simulink library "alphaBetaLE_ul"  (R2020a)
settings: Solver=VariableStepAuto  StartTime=0.0  StopTime=10.0  RelTol=1e-3
libraries: vrlib x1, vectorNormalizer_ul x1
settings Model: Creator=mcobb  LastModifiedBy=John Jr
settings DataIOCC: ReturnWorkspaceOutputs=off
settings DebuggingCC: ArithmeticOperatorsInVariantConditions=warning
settings SFSimCC: CustomCodeUndefinedFunction=UseInterfaceOnly

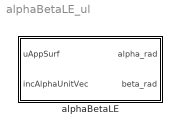
== system alphaBetaLE_ul ==
  alphaBetaLE : Subsystem  TreatAsAtomicUnit=on
      settings: MinAlgLoopOccurrences=on

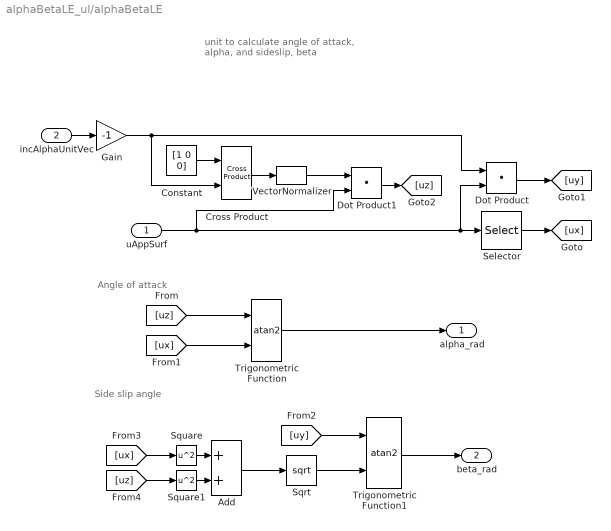
== system alphaBetaLE_ul/alphaBetaLE ==
  note: Side slip angle
  note: Angle of attack
  note: unit to calculate angle of attack,
      | alpha, and sideslip, beta
  uAppSurf : Inport
  incAlphaUnitVec : Inport  Port=2
  Add : Sum
  Constant : Constant  Value=[1 0 0]
  Cross Product : vrlib/Utilities/Cross Product
  Dot Product : DotProduct  InputSameDT=on  OutDataTypeStr=Inherit: Inherit via internal rule
  Dot Product1 : DotProduct  InputSameDT=on  OutDataTypeStr=Inherit: Inherit via internal rule
  Gain : Gain  Gain=-1
  Selector : Selector  InputPortWidth=3  IndexOptions=Index vector (dialog)  Indices=1  OutputSizes=1
  Sqrt : Sqrt  SaturateOnIntegerOverflow=on
  Square : Math  Operator=square  SignedPower=on  SaturateOnIntegerOverflow=on
  Square1 : Math  Operator=square  SignedPower=on  SaturateOnIntegerOverflow=on
  Trigonometric Function : Trigonometry  Operator=atan2
  Trigonometric Function1 : Trigonometry  Operator=atan2
  "VectorNormalizer " : vectorNormalizer_ul/VectorNormalizer   SystemSampleTime=-1  Latency=0  AutoFrameSizeCalculation=off
  alpha_rad : Outport  VectorParamsAs1DForOutWhenUnconnected=off
  beta_rad : Outport  Port=2  VectorParamsAs1DForOutWhenUnconnected=off
  wires:
  Dot Product1/1 -> [uz]
  Square/1 -> Add/1
  Square1/1 -> Add/2
  Add/1 -> Sqrt/1
  [uz] -> Square1/1
  [ux] -> Square/1
  Trigonometric Function/1 -> alpha_rad/1
  Trigonometric Function1/1 -> beta_rad/1
  [uz] -> Trigonometric Function/1
  [ux] -> Trigonometric Function/2
  [uy] -> Trigonometric Function1/1
  Sqrt/1 -> Trigonometric Function1/2
  Cross Product/1 -> "VectorNormalizer "/1
  uAppSurf/1 -> Dot Product/2, Selector/1, Dot Product1/2
  "VectorNormalizer "/1 -> Dot Product1/1
  Dot Product/1 -> [uy]
  Selector/1 -> [ux]
  Constant/1 -> Cross Product/1
  incAlphaUnitVec/1 -> Gain/1
  Gain/1 -> Cross Product/2, Dot Product/1
